simulink library "MIL_Test"  (Simulink 7.0)
values from neighbouring files (symbols this model uses):
  TID = min('TI' == AFT(1:2))    [PAS_callback.m]    (also in PSTID_callback.m = [block '/TID'])
undefined symbols (not defined in the file or in its folder): getdatatypespecs, slcm, StepSize
libraries: simulink x71, MIL_Test x6
(part 4 of 11)

== system MIL_Test/Validation Function/Feature extraction/Time @ sig = x/Relative tolerance ==
  sig : Inport  OutDataType=sfix(16)  OutScaling=2^0
  ref : Inport  Port=2  OutDataType=sfix(16)  OutScaling=2^0
  Abs : Abs
  Abs1 : Abs
  Add : Sum  Inputs=+-  OutDataType=sfix(16)  OutScaling=2^-10
  Divide1 : Product  Inputs=**/  OutDataType=sfix(16)  OutScaling=2^-10
  Max : Constant  Value=100  OutDataType=sfix(16)  OutScaling=2^0
  Relational Operator : RelationalOperator  Operator=<=  LogicOutDataTypeMode=boolean
  Relative Tolerance : Constant  Value=0.0001  OutDataType=sfix(16)  OutScaling=2^0
  sig == ref : Outport  OutDataType=sfix(16)  OutScaling=2^0
  wires:
  Abs1/1 -> Divide1/1
  Relational Operator/1 -> sig == ref/1
  Relative Tolerance/1 -> Divide1/2
  Max/1 -> Divide1/3
  Divide1/1 -> Relational Operator/2
  ref/1 -> Abs1/1, Add/2
  sig/1 -> Add/1
  Add/1 -> Abs/1
  Abs/1 -> Relational Operator/1

== system MIL_Test/Validation Function/Feature extraction/Time since signal constant/Detect constant ==
  Signal : Inport  OutDataType=sfix(16)  OutScaling=2^0
  Clock : Clock
      settings: Decimation=10
  Constant1 : Constant  Value=0  OutDataTypeMode=boolean  OutDataType=sfix(16)  OutScaling=2^0
  Memory : Memory
  Relative tolerance : Subsystem
  Switch : Switch  Criteria=u2 > Threshold
  Constant : Outport  OutDataType=sfix(16)  OutScaling=2^0
  wires:
  Switch/1 -> Constant/1
  Relative tolerance/1(sig == ref) -> Switch/1
  Clock/1 -> Switch/2
  Constant1/1 -> Switch/3
  Memory/1 -> Relative tolerance/2(ref)
  Signal/1 -> Relative tolerance/1(sig), Memory/1

== system MIL_Test/Validation Function/TODO/<system name>/<Requirement name> ==
  InOut Bus : Inport  OutDataType=sfix(16)  OutScaling=2^0
  <Assertions name> : Subsystem  Description=Assertions template. Create a new assertions block from this template.
  <Preconditions name> : Subsystem  Description=Preconditions template. Create new preconditions blocks using this template.
  Bus Creator : BusCreator  Inputs=1
  Test Info : Outport  OutDataType=sfix(16)  OutScaling=2^0
  wires:
  <Preconditions name>/1(Activate) -> <Assertions name>/1(Precond)
  Bus Creator/1 -> Test Info/1
  <Assertions name>/1(VF info) -> Bus Creator/1
  InOut Bus/1 -> <Preconditions name>/1(InOut Bus), <Assertions name>/2(InOut Bus)

== system MIL_Test/Validation Function/TODO/Assertions/Fault info ==
  Local Verdict : Inport  OutDataType=sfix(16)  OutScaling=2^0
  Expected lower limit : Inport  Port=2  OutDataType=sfix(16)  OutScaling=2^0
  Expected upper limit : Inport  Port=3  OutDataType=sfix(16)  OutScaling=2^0
  Actual Data : Inport  Port=4  OutDataType=sfix(16)  OutScaling=2^0
  Enable : EnablePort
  Assertions : Constant  Value=Ass  OutDataType=sfix(16)  OutScaling=2^0
  Bus Creator : BusCreator  Inputs=5
  Bus Creator1 : BusCreator  Inputs=3
  Data Type Conversion{,1..3} (4 alike) : DataTypeConversion  OutDataType=sfix(16)  OutScaling=2^0
  Preconditions : Constant  Value=Pre  OutDataType=sfix(16)  OutScaling=2^0
  Requirement : Constant  Value=Req  OutDataType=sfix(16)  OutScaling=2^0
  VF info : Outport  OutDataType=sfix(16)  OutScaling=2^0  OutputWhenDisabled=reset  InitialOutput=[2]
  wires:
  Requirement/1 -> Bus Creator1/3  "Requirement"
  Preconditions/1 -> Bus Creator1/2  "Preconditions"
  Assertions/1 -> Bus Creator1/1  "Assertions"
  Data Type Conversion3/1 -> Bus Creator/4  "Actual data"
  Data Type Conversion2/1 -> Bus Creator/3  "Expected upper limit"
  Data Type Conversion1/1 -> Bus Creator/2  "Expected lower limit"
  Data Type Conversion/1 -> Bus Creator/1  "Local verdict"
  Local Verdict/1 -> Data Type Conversion/1  "Local verdict"
  Expected upper limit/1 -> Data Type Conversion2/1  "Expected upper limit"
  Expected lower limit/1 -> Data Type Conversion1/1  "Expected lower limit"
  Actual Data/1 -> Data Type Conversion3/1  "Actual Data"
  Bus Creator1/1 -> Bus Creator/5  "Source"
  Bus Creator/1 -> VF info/1

== system MIL_Test/Validation Function/TODO/Assertions/Signal comparison ==
  Bound : Subsystem  mask(Bound){cm=>=, Lower=0, Upper=1}
      mask prompts: cm "Comparison method:"; Upper "Mask Parameter 3:"
      mask help:
      | Compare a signal with a reference using the specified comparison method.
      |
      | Output verdict V and lower (LL) and upper (UL) limits for reporting.
      |
      | For '==' or '~=' use "Range - Gap"
      mask init:
      | set_param([get_param(gcb,'Parent') '/' get_param(gcb,'Name') '/Relational Operator'],'Operator',get_param(gcb,'cm'));
      | set_param(gcb,'Upper',num2str(uint8(max(get_param([get_param(gcb,'Parent') '/' get_param(gcb,'Name') '/Relational Operator'],'Operator') == '>'))));
      | set_param(gcb,'Lower',num2str(uint8(max(get_param([get_param(gcb,'Parent') '/' get_param(gcb,'Name') '/Relational Operator'],'Operator') == '<'))));
      mask StyleString: popup(>|>=|<=|<),edit,edit
      mask Display:
      | port_label('output', 1, 'V');
      | port_label('output', 2, 'LL');
      | port_label('output', 3, 'UL');
      | port_label('input', 1, 'Sig');
      | port_label('input', 2, 'Ref');
      | text(0.05,0.5,get_param(get_param([get_param(gcb,'Parent') '/' get_param(gcb,'Name') '/Relational Operator'],'handle'),'Operator'));
  Range - Gap Absolute tolerance : Subsystem  mask(Range - Gap Absolute Tolerance){GorR=Range, AbsoluteTolerance=100}
      mask prompts: GorR "Use range or gap"; AbsoluteTolerance "Absolute Tolerance"
      mask help:
      | Check that a signal stays inside a range or outside a gap around a reference signal. Specify the range or the gap absolute to the reference signal.
      |
      | Output verdict V and lower (LL) and upper (UL) limits for reporting.
      mask init: same as MIL_Test/Test Data/Signal comparison/Range - Gap Relative tolerance Precond
      mask StyleString: popup(Range|Gap  ),edit
      mask Display:
      | port_label('output',1,'V');
      | port_label('output',2,'LL');
      | port_label('output',3,'UL');
      | port_label('input',1,'Sig');
      | port_label('input',2,'Ref');
      | text(0.40,0.53,'+');
      | text(0.415,0.46,'-');
      | text(0.5,0.5,num2str(AbsoluteTolerance));
      | text(0.05,0.5,helpVariable2);
  Range - Gap Relative tolerance : Subsystem  mask(Range - Gap Relative Tolerance){GorR=Range, RelativeTolerance=1}
      mask prompts: GorR "Use range or gap"; RelativeTolerance "Relative Tolerance in Percent"
      mask help:
      | Check that a signal stays inside a range or outside a gap around a reference signal. Specify the range or the gap relative to the reference signal.
      |
      | Output verdict V and lower (LL) and upper (UL) limits for reporting.
      mask init: same as MIL_Test/Test Data/Signal comparison/Range - Gap Relative tolerance Precond
      mask StyleString: popup(Range|Gap  ),edit
      mask Display:
      | port_label('output',1,'V');
      | port_label('output',2,'LL');
      | port_label('output',3,'UL');
      | port_label('input',1,'Sig');
      | port_label('input',2,'Ref');
      | text(0.425,0.5,[num2str(RelativeTolerance) ' %']);
      | text(0.05,0.5,helpVariable2);
  Range - Gap Tolerance range : Subsystem  mask(Range - Gap Tolerance range){GorR=Range}
      mask prompts: GorR "Use range or gap"
      mask help:
      | Check that a signal stays inside a dynamically specified value range.
      |
      | Output verdict V and lower (LL) and upper (UL) limits for reporting.
      mask init:
      | if max(get_param(gcb,'GorR') == ' ') % Gap
      |     helpVariable1 = '<=';
      | else % Range
      |     helpVariable1 = '>=';
      | end
      | set_param([get_param(gcb,'Parent') '/' get_param(gcb,'Name') '/Relational Operator'],'Operator',helpVariable1);
      | clear helpVariable1;
      mask StyleString: popup(Range|Gap  )
      mask Display:
      | port_label('output',1,'V');
      | port_label('output',2,'LL');
      | port_label('output',3,'UL');
      | port_label('input',1,'Sig');
      | port_label('input',2,'Lower Bound');
      | port_label('input',3,'Upper Bound');
      | patch(0.05+[0.3 0.7 0.7 0.3],-0.05+[0.8 0.8 0.9 0.9],[1 1 1]*double(not(max(get_param(gcb,'GorR') == ' '))));
      | patch(0.05+[0.3 0.7 0.7 0.3],-0.05+[0.9 0.9 0.95 0.95],[1 1 1]*double(max(get_param(gcb,'GorR') == ' ')));
      | patch(0.05+[0.3 0.7 0.7 0.3],-0.05+[0.75 0.75 0.8 0.8],[1 1 1]*double(max(get_param(gcb,'GorR') == ' ')));
      | patch(0.05+[0.25 0.25 0.8 0.8 0.26 0.26],[0.95 0.65 0.65 0.66 0.66 0.95],[0 0 0]);
      | patch(0.033+[0.27 0.22 0.23 0.27 0.31 0.32 0.27],0.02+[0.95 0.85 0.85 0.89 0.85 0.85 0.95],[0 0 0]);
      | patch(0.17+[0.7 0.6 0.6 0.65 0.6 0.6 0.7],-0.043+[0.7 0.63 0.64 0.7 0.76 0.77 0.7],[0 0 0]);

== system MIL_Test/Validation Function/TODO/Model Info/EmptySubsystem ==

== system MIL_Test/Validation Function/TODO/Preconditions/Signal comparison ==
  Bound : Subsystem  mask(Bound){cm=>=}
      mask prompts: cm "Comparison method:"
      mask help:
      | Compare a signal with a reference using the specified comparison method.
      |
      | For '==' or '~=' use "Range - Gap"
      mask init:
      | bp = get_param(gcbh,'Parent');
      | bn = get_param(gcbh,'Name');
      | set_param([bp '/' bn '/RelOp'],'Operator',get_param(gcbh,'cm'));
      mask StyleString: popup(>|>=|<=|<)
      mask Display:
      | port_label('output', 1, 'A');
      | port_label('input', 1, 'Sig');
      | port_label('input', 2, 'Ref');
      | text(0.05,0.5,get_param(get_param([get_param(gcb,'Parent') '/' get_param(gcb,'Name') '/RelOp'],'handle'),'Operator'));
  Range - Gap Absolute tolerance : Subsystem  mask(Range - Gap Absolute Tolerance){GorR=Range, AbsoluteTolerance=100}
      mask prompts: GorR "Use range or gap"; AbsoluteTolerance "Absolute Tolerance"
      mask help: Check that a signal stays inside a range or outside a gap around a reference signal. Specify the range or the gap absolute to the reference signal.
      mask init:
      | if max(get_param(gcb,'GorR') == ' ') % Gap
      |     helpVariable1 = '>=';
      |     helpVariable2 = '~=';
      | else % Range
      |     helpVariable1 = '<=';
      |     helpVariable2 = '==';
      | end
      | set_param([get_param(gcb,'Parent') '/' get_param(gcb,'Name') '/Relational Operator'],'Operator',helpVariable1);
      | set_param(gcb,'Op',helpVariable2);
      | clear helpVariable1;
      mask StyleString: popup(Range|Gap  ),edit
      mask Display:
      | port_label('output',1,'A');
      | port_label('input',1,'Sig');
      | port_label('input',2,'Ref');
      | text(0.40,0.53,'+');
      | text(0.415,0.46,'-');
      | text(0.5,0.5,num2str(AbsoluteTolerance));
      | text(0.05,0.5,helpVariable2);
  Range - Gap Relative tolerance : Subsystem  mask(Range - Gap Relative Tolerance){GorR=Range, RelativeTolerance=1}
      mask prompts: GorR "Use range or gap"; RelativeTolerance "Relative Tolerance in Percent"
      mask help: Check that a signal stays inside a range or outside a gap around a reference signal. Specify the range or the gap relative to the reference signal.
      mask init: same as MIL_Test/Test Data/Signal comparison/Range - Gap Relative tolerance Precond
      mask StyleString: popup(Range|Gap  ),edit
      mask Display:
      | port_label('output',1,'A');
      | port_label('input',1,'Sig');
      | port_label('input',2,'Ref');
      | text(0.425,0.5,[num2str(RelativeTolerance) ' %']);
      | text(0.05,0.5,helpVariable2);
  Range - Gap Tolerance range : Subsystem  mask(Range - Gap Tolerance range){GorR=Range}
      mask prompts: GorR "Use range or gap"
      mask help: Check that a signal stays inside a dynamically specified value range.
      mask init: same as MIL_Test/Validation Function/TODO/Assertions/Signal comparison/Range - Gap Tolerance range
      mask StyleString: popup(Range|Gap  )
      mask Display:
      | port_label('output',1,'A');
      | port_label('input',1,'Sig');
      | port_label('input',2,'Lower Bound');
      | port_label('input',3,'Upper Bound');
      | patch(0.05+[0.3 0.7 0.7 0.3],-0.05+[0.8 0.8 0.9 0.9],[1 1 1]*double(not(max(get_param(gcb,'GorR') == ' '))));
      | patch(0.05+[0.3 0.7 0.7 0.3],-0.05+[0.9 0.9 0.95 0.95],[1 1 1]*double(max(get_param(gcb,'GorR') == ' ')));
      | patch(0.05+[0.3 0.7 0.7 0.3],-0.05+[0.75 0.75 0.8 0.8],[1 1 1]*double(max(get_param(gcb,'GorR') == ' ')));
      | patch(0.05+[0.25 0.25 0.8 0.8 0.26 0.26],[0.95 0.65 0.65 0.66 0.66 0.95],[0 0 0]);
      | patch(0.033+[0.27 0.22 0.23 0.27 0.31 0.32 0.27],0.02+[0.95 0.85 0.85 0.89 0.85 0.85 0.95],[0 0 0]);
      | patch(0.17+[0.7 0.6 0.6 0.65 0.6 0.6 0.7],-0.043+[0.7 0.63 0.64 0.7 0.76 0.77 0.7],[0 0 0]);

== system MIL_Test/Validation Function/TODO/Validation FunctionsTemplate/Arbitration ==
  In1 : Inport  OutDataType=sfix(16)  OutScaling=2^0
  Collect Verdicts : MinMax  Inputs=3  OutDataType=sfix(16)  OutScaling=2^0
  Memory : Memory  Orientation=left  X0=2
  Out1 : Outport  OutDataType=sfix(16)  OutScaling=2^0
  wires:
  Collect Verdicts/1 -> Memory/1, Out1/1
  In1/1 -> Collect Verdicts/1
  Memory/1 -> Collect Verdicts/3

== system MIL_Test/Validation Function/TODO/Validation FunctionsTemplate/Datatype conversion ==
  InOutBus : Inport  OutDataType=sfix(16)  OutScaling=2^0
  Bus Creator{,1..5} (6 alike) : BusCreator  Inputs=2
  Bus Selector : BusSelector  OutputSignals=Inputs,Outputs
  Bus Selector1 : BusSelector  OutputSignals=v_Fzg,signal2
  Bus Selector2 : BusSelector  OutputSignals=signal1,signal2
  Bus Selector3 : BusSelector  OutputSignals=phi_Acc,phi_Brake
  Bus Selector4 : BusSelector  OutputSignals=T_des_Drive,T_des_Brake
  Bus Selector5 : BusSelector  OutputSignals=AccPedal,BrakePedal
  Data Type Conversion{,1..6} (7 alike) : DataTypeConversion  OutDataType=sfix(16)  OutScaling=2^0
  InOut Bus : Outport  OutDataType=sfix(16)  OutScaling=2^0
  wires:
  Bus Creator5/1 -> InOut Bus/1  "InOutBus"
  Bus Creator4/1 -> Bus Creator5/2  "Outputs"
  Bus Creator3/1 -> Bus Creator5/1  "Inputs"
  Bus Creator1/1 -> Bus Creator4/2
  Bus Creator/1 -> Bus Creator4/1
  Data Type Conversion/1 -> Bus Creator3/1  "v_Fzg"
  Bus Creator2/1 -> Bus Creator3/2  "signal2"
  Data Type Conversion2/1 -> Bus Creator2/2  "phi_Brake"
  Data Type Conversion1/1 -> Bus Creator2/1  "phi_Acc"
  Data Type Conversion6/1 -> Bus Creator1/2  "BrakePedal"
  Data Type Conversion5/1 -> Bus Creator1/1  "AccPedal"
  Data Type Conversion4/1 -> Bus Creator/2  "T_des_Brake"
  Data Type Conversion3/1 -> Bus Creator/1  "T_des_Drive"
  Bus Selector5/2 -> Data Type Conversion6/1  "<BrakePedal>"
  Bus Selector5/1 -> Data Type Conversion5/1  "<AccPedal>"
  Bus Selector4/2 -> Data Type Conversion4/1  "<T_des_Brake>"
  Bus Selector4/1 -> Data Type Conversion3/1  "<T_des_Drive>"
  Bus Selector3/2 -> Data Type Conversion2/1  "<phi_Brake>"
  Bus Selector3/1 -> Data Type Conversion1/1  "<phi_Acc>"
  Bus Selector1/1 -> Data Type Conversion/1  "<v_Fzg>"
  Bus Selector2/2 -> Bus Selector5/1  "<signal2>"
  Bus Selector2/1 -> Bus Selector4/1  "<signal1>"
  Bus Selector1/2 -> Bus Selector3/1  "<signal2>"
  Bus Selector/2 -> Bus Selector2/1  "<Outputs>"
  Bus Selector/1 -> Bus Selector1/1  "<Inputs>"
  InOutBus/1 -> Bus Selector/1

== system MIL_Test/Validation Function/TODO/Validation FunctionsTemplate/Requirement ==
  InOut Bus : Inport  OutDataType=sfix(16)  OutScaling=2^0
  Assertions : Subsystem  TreatAsAtomicUnit=on
  Bus Creator : BusCreator  Inputs=1
  Preconditions : Subsystem
  Validation Information : Outport  OutDataType=sfix(16)  OutScaling=2^0
  wires:
  Assertions/1(VF info) -> Bus Creator/1
  Bus Creator/1 -> Validation Information/1
  InOut Bus/1 -> Preconditions/1(InOut Bus), Assertions/2(InOut Bus)
  Preconditions/1(Activate) -> Assertions/1(Activate)

== system MIL_Test/Validation Function/TODO/Validation FunctionsTemplate/Requirement2 ==
  InOut Bus : Inport  OutDataType=sfix(16)  OutScaling=2^0
  Assertions : Subsystem  TreatAsAtomicUnit=on
  Bus Creator : BusCreator  Inputs=1
  Preconditions : Subsystem
  Validation Information : Outport  OutDataType=sfix(16)  OutScaling=2^0
  wires:
  Preconditions/1(Activate) -> Assertions/1(Activate)
  InOut Bus/1 -> Assertions/2(InOut Bus), Preconditions/1(InOut Bus)
  Bus Creator/1 -> Validation Information/1
  Assertions/1(VF info) -> Bus Creator/1

== system MIL_Test/Validation Function/Test Evaluation Architecture/<system name>/<Requirement name> ==
  InOut Bus : Inport  OutDataType=sfix(16)  OutScaling=2^0
  <Assertions name> : Subsystem  Description=Assertions template. Create a new assertions block from this template.
  <Preconditions name> : Subsystem  Description=Preconditions template. Create new preconditions blocks using this template.
  Bus Creator : BusCreator  Inputs=1
  Test Info : Outport  OutDataType=sfix(16)  OutScaling=2^0
  wires:
  InOut Bus/1 -> <Assertions name>/2(InOut Bus), <Preconditions name>/1(InOut Bus)
  <Assertions name>/1(VF info) -> Bus Creator/1
  Bus Creator/1 -> Test Info/1
  <Preconditions name>/1(Activate) -> <Assertions name>/1(Precond)

== system MIL_Test/Validation Function/Test Evaluation Architecture/<system name>/Arbitration ==
  In1 : Inport  OutDataType=sfix(16)  OutScaling=2^0
  Collect Verdicts : MinMax  Inputs=2  OutDataType=sfix(16)  OutScaling=2^0
  Memory : Memory  Orientation=left  X0=2
  Out1 : Outport  OutDataType=sfix(16)  OutScaling=2^0
  wires:
  Memory/1 -> Collect Verdicts/2
  Collect Verdicts/1 -> Memory/1, Out1/1
  In1/1 -> Collect Verdicts/1

== system MIL_Test/Test Control/Test Control Architecture/Connection Helpers/TestControl for  TestCases Sequencing NoMask/IF Signal@SimStopTime for TC = value1 ==
  Signal : Inport  OutDataType=sfix(16)  OutScaling=2^0
  Current Sim StopTime : Constant  Value=currentStopTime  OutDataType=sfix(16)  OutScaling=2^0
  If : If  IfExpression=u1 ~= 1
  Model Info : simulink/Model-Wide Utilities/Model Info  SystemSampleTime=-1  InitialBlockCM=None  BlockCM=None  Frame=on  DisplayStringWithTags=|  HorizontalTextAlignment=Center  LeftAlignmentValue=0.5  SourceBlockDiagram=MIL_Test  TagMaxNumber=20
      | Flag Fullfillment = 1, then condition is true 
      | Flag Fullfillment = 0, then condition is false
  if Signal@t for TC = pass : Subsystem
  "if false, then  TC4 for 200" : Subsystem
  "if true, then  TC2 for 400" : Subsystem
  Fulfillment : Outport  OutDataType=sfix(16)  OutScaling=2^0
  wires:
  Current Sim StopTime/1 -> if Signal@t for TC = pass/1(@time)
  Signal/1 -> if Signal@t for TC = pass/2(Signal1)
  If/1 -> "if false, then  TC4 for 200"/Action
  If/2 -> "if true, then  TC2 for 400"/Action
  if Signal@t for TC = pass/1(Control Seq1) -> Fulfillment/1

== system MIL_Test/Test Control/Test Control Architecture/Connection Helpers/TestControl for  TestCases Sequencing NoMask/IF signal @[timeUp, timeDown] for TC = value1 ==
  Signal : Inport  OutDataType=sfix(16)  OutScaling=2^0
  TimeDown : Constant  Value=timeDown  OutDataType=sfix(16)  OutScaling=2^0
  TimeUp : Constant  Value=timeUp  OutDataType=sfix(16)  OutScaling=2^0
  if Signal@ [TDown,TUp]  for TC = Value : Subsystem
  Fulfillment : Outport  OutDataType=sfix(16)  OutScaling=2^0
  wires:
  TimeDown/1 -> if Signal@ [TDown,TUp]  for TC = Value/1(@timeDown)
  TimeUp/1 -> if Signal@ [TDown,TUp]  for TC = Value/2(@timeUp)
  Signal/1 -> if Signal@ [TDown,TUp]  for TC = Value/3(Signal)
  if Signal@ [TDown,TUp]  for TC = Value/1(Control Seq) -> Fulfillment/1

== system MIL_Test/Test Control/Test Control Architecture/Connection Helpers/TestControl for  TestCases Sequencing NoMask/IF signal@time for TC = value1 ==
  Signal : Inport  OutDataType=sfix(16)  OutScaling=2^0
  given Time : Constant  Value=time  OutDataType=sfix(16)  OutScaling=2^0
  if Signal@t for TC = pass : Subsystem
  Fulfillment : Outport  OutDataType=sfix(16)  OutScaling=2^0
  wires:
  given Time/1 -> if Signal@t for TC = pass/1(@time)
  Signal/1 -> if Signal@t for TC = pass/2(Signal1)
  if Signal@t for TC = pass/1(Control Seq) -> Fulfillment/1

== system MIL_Test/Test Control/Test Control Architecture/Test Control Conditions/IF Signal@SimStopTime for TC = value1/if Signal@t for TC = pass ==
  @time : Inport  OutDataType=sfix(16)  OutScaling=2^0
  Signal1 : Inport  Port=2  OutDataType=sfix(16)  OutScaling=2^0
  ClockAtEnd : Clock
      settings: Decimation=10
  Relational Operator1 : RelationalOperator  LogicOutDataTypeMode=boolean
  check in range : Subsystem  TreatAsAtomicUnit=on
  Control Seq1 : Outport  OutDataType=sfix(16)  OutScaling=2^0
  wires:
  Relational Operator1/1 -> check in range/Enable, check in range/1(@[time])
  check in range/1(Control Seq) -> Control Seq1/1
  Signal1/1 -> check in range/2(Signal)
  @time/1 -> Relational Operator1/2
  ClockAtEnd/1 -> Relational Operator1/1

== system MIL_Test/Test Control/Test Control Architecture/Test Control Conditions/IF Signal@SimStopTime for TC = value1/if false, then  TC4 for 200 ==
  Action Port : ActionPort
  Embedded MATLAB Function : Stateflow chart

== system MIL_Test/Test Control/Test Control Architecture/Test Control Conditions/IF Signal@SimStopTime for TC = value1/if true, then  TC2 for 400 ==
  Action Port : ActionPort
  Embedded MATLAB Function : Stateflow chart

== system MIL_Test/Test Control/Test Control Architecture/Test Control Conditions/IF signal @[timeUp, timeDown] for TC = value1/if Signal@ [TDown,TUp]  for TC = Value ==
  @timeDown : Inport  OutDataType=sfix(16)  OutScaling=2^0
  @timeUp : Inport  Port=2  OutDataType=sfix(16)  OutScaling=2^0
  Signal : Inport  Port=3  OutDataType=sfix(16)  OutScaling=2^0
  ClockDuring : Clock
      settings: Decimation=10
  Logical Operator1 : Logic  AllPortsSameDT=off  OutDataTypeMode=boolean
  Relational Operator1 : RelationalOperator  LogicOutDataTypeMode=boolean
  Relational Operator2 : RelationalOperator  Operator=<=  LogicOutDataTypeMode=boolean
  check in range : Subsystem  TreatAsAtomicUnit=on
  Control Seq : Outport  OutDataType=sfix(16)  OutScaling=2^0
  wires:
  check in range/1(Control Seq) -> Control Seq/1
  Signal/1 -> check in range/2(Signal)
  Logical Operator1/1 -> check in range/Enable, check in range/1(@[time])
  Relational Operator2/1 -> Logical Operator1/2
  Relational Operator1/1 -> Logical Operator1/1
  @timeUp/1 -> Relational Operator2/2
  @timeDown/1 -> Relational Operator1/2
  ClockDuring/1 -> Relational Operator2/1, Relational Operator1/1

== system MIL_Test/Test Control/Test Control Architecture/Test Control Conditions/IF signal@time for TC = value1/if Signal@t for TC = pass ==
  @time : Inport  OutDataType=sfix(16)  OutScaling=2^0
  Signal1 : Inport  Port=2  OutDataType=sfix(16)  OutScaling=2^0
  ClockAtTime : Clock
      settings: Decimation=10
  Relational Operator1 : RelationalOperator  LogicOutDataTypeMode=boolean
  check in range : Subsystem  TreatAsAtomicUnit=on
  Control Seq : Outport  OutDataType=sfix(16)  OutScaling=2^0
  wires:
  check in range/1(Control Seq) -> Control Seq/1
  Signal1/1 -> check in range/2(Signal)
  Relational Operator1/1 -> check in range/Enable, check in range/1(@[time])
  @time/1 -> Relational Operator1/2
  ClockAtTime/1 -> Relational Operator1/1

== system MIL_Test/Test Control/Test Control Architecture/Test Control Conditions/IF signal@time1/if Signal@t for TC = pass ==
  @time : Inport  OutDataType=sfix(16)  OutScaling=2^0
  Signal1 : Inport  Port=2  OutDataType=sfix(16)  OutScaling=2^0
  Clock : Clock
      settings: Decimation=10
  Relational Operator1 : RelationalOperator  LogicOutDataTypeMode=boolean
  check in range : Subsystem  TreatAsAtomicUnit=on
  Control Seq : Outport  OutDataType=sfix(16)  OutScaling=2^0
  wires:
  Relational Operator1/1 -> check in range/Enable, check in range/1(@[time])
  check in range/1(Control Seq) -> Control Seq/1
  Signal1/1 -> check in range/2(Signal)
  @time/1 -> Relational Operator1/2
  Clock/1 -> Relational Operator1/1

== system MIL_Test/Test Control/Test Control Architecture/Test Control Conditions/IF signal@time1/if false, then  TC4 for 200 ==
  Action Port : ActionPort
  Embedded MATLAB Function : Stateflow chart

== system MIL_Test/Test Control/Test Control Architecture/Test Control Conditions/IF signal@time1/if true, then  TC2 for 400 ==
  Action Port : ActionPort
  Embedded MATLAB Function : Stateflow chart

== system MIL_Test/Test Data/Feature generation/Generate  local maximum  with given slope/Limited Ramp Increasing/Enabled Subsystem1 ==
  In2 : Inport  OutDataType=sfix(16)  OutScaling=2^0
  Enable : EnablePort  StatesWhenEnabling=reset
  MaxValue1 : Outport  OutDataType=sfix(16)  OutScaling=2^0  InitialOutput=[0]
  wires:
  In2/1 -> MaxValue1/1

== system MIL_Test/Test Data/Feature generation/Generate timed limited decrease/Subsystem/Subsystem1 ==
  In1 : Inport  OutDataType=sfix(16)  OutScaling=2^0
  In2 : Inport  Port=2  OutDataType=sfix(16)  OutScaling=2^0
  In3 : Inport  Port=3  OutDataType=sfix(16)  OutScaling=2^0
  Output1 : Sum  Inputs=|+-+  OutDataType=sfix(16)  OutScaling=2^0  SaturateOnIntegerOverflow=on  InputSameDT=on
  RO : RelationalOperator  Operator=<  LogicOutDataTypeMode=boolean
  Switch : Switch  Criteria=u2 > Threshold
  Out1 : Outport  OutDataType=sfix(16)  OutScaling=2^0
  wires:
  In3/1 -> Output1/3
  Output1/1 -> Switch/1
  RO/1 -> Switch/2
  Switch/1 -> Out1/1
  In2/1 -> RO/1, Output1/1, Switch/3  "U(k)"
  In1/1 -> RO/2, Output1/2

== system MIL_Test/Test Data/Feature generation/Generate timed limited decrease/Subsystem/Subsystem10 ==
  In1 : Inport  OutDataType=sfix(16)  OutScaling=2^0
  In2 : Inport  Port=2  OutDataType=sfix(16)  OutScaling=2^0
  In3 : Inport  Port=3  OutDataType=sfix(16)  OutScaling=2^0
  Output1 : Sum  Inputs=|+-+  OutDataType=sfix(16)  OutScaling=2^0  SaturateOnIntegerOverflow=on  InputSameDT=on
  RO : RelationalOperator  Operator=<  LogicOutDataTypeMode=boolean
  Switch : Switch  Criteria=u2 > Threshold
  Out1 : Outport  OutDataType=sfix(16)  OutScaling=2^0
  wires:
  In3/1 -> Output1/3
  Output1/1 -> Switch/1
  RO/1 -> Switch/2
  Switch/1 -> Out1/1
  In2/1 -> RO/1, Output1/1, Switch/3  "U(k)"
  In1/1 -> RO/2, Output1/2

== system MIL_Test/Test Data/Feature generation/Generate timed limited decrease/Subsystem/Subsystem11 ==
  In1 : Inport  OutDataType=sfix(16)  OutScaling=2^0
  In2 : Inport  Port=2  OutDataType=sfix(16)  OutScaling=2^0
  In3 : Inport  Port=3  OutDataType=sfix(16)  OutScaling=2^0
  Output1 : Sum  Inputs=|+-+  OutDataType=sfix(16)  OutScaling=2^0  SaturateOnIntegerOverflow=on  InputSameDT=on
  RO : RelationalOperator  Operator=<  LogicOutDataTypeMode=boolean
  Switch : Switch  Criteria=u2 > Threshold
  Out1 : Outport  OutDataType=sfix(16)  OutScaling=2^0
  wires:
  In3/1 -> Output1/3
  Output1/1 -> Switch/1
  RO/1 -> Switch/2
  Switch/1 -> Out1/1
  In2/1 -> RO/1, Output1/1, Switch/3  "U(k)"
  In1/1 -> RO/2, Output1/2

== system MIL_Test/Test Data/Feature generation/Generate timed limited decrease/Subsystem/Subsystem12 ==
  In1 : Inport  OutDataType=sfix(16)  OutScaling=2^0
  In2 : Inport  Port=2  OutDataType=sfix(16)  OutScaling=2^0
  In3 : Inport  Port=3  OutDataType=sfix(16)  OutScaling=2^0
  Output1 : Sum  Inputs=|+-+  OutDataType=sfix(16)  OutScaling=2^0  SaturateOnIntegerOverflow=on  InputSameDT=on
  RO : RelationalOperator  Operator=<  LogicOutDataTypeMode=boolean
  Switch : Switch  Criteria=u2 > Threshold
  Out1 : Outport  OutDataType=sfix(16)  OutScaling=2^0
  wires:
  In3/1 -> Output1/3
  Output1/1 -> Switch/1
  RO/1 -> Switch/2
  Switch/1 -> Out1/1
  In2/1 -> RO/1, Output1/1, Switch/3  "U(k)"
  In1/1 -> RO/2, Output1/2

== system MIL_Test/Test Data/Feature generation/Generate timed limited decrease/Subsystem/Subsystem13 ==
  In1 : Inport  OutDataType=sfix(16)  OutScaling=2^0
  In2 : Inport  Port=2  OutDataType=sfix(16)  OutScaling=2^0
  In3 : Inport  Port=3  OutDataType=sfix(16)  OutScaling=2^0
  Output1 : Sum  Inputs=|+-+  OutDataType=sfix(16)  OutScaling=2^0  SaturateOnIntegerOverflow=on  InputSameDT=on
  RO : RelationalOperator  Operator=<  LogicOutDataTypeMode=boolean
  Switch : Switch  Criteria=u2 > Threshold
  Out1 : Outport  OutDataType=sfix(16)  OutScaling=2^0
  wires:
  In3/1 -> Output1/3
  Output1/1 -> Switch/1
  RO/1 -> Switch/2
  Switch/1 -> Out1/1
  In2/1 -> RO/1, Output1/1, Switch/3  "U(k)"
  In1/1 -> RO/2, Output1/2

== system MIL_Test/Test Data/Feature generation/Generate timed limited decrease/Subsystem/Subsystem14 ==
  In1 : Inport  OutDataType=sfix(16)  OutScaling=2^0
  In2 : Inport  Port=2  OutDataType=sfix(16)  OutScaling=2^0
  In3 : Inport  Port=3  OutDataType=sfix(16)  OutScaling=2^0
  Output1 : Sum  Inputs=|+-+  OutDataType=sfix(16)  OutScaling=2^0  SaturateOnIntegerOverflow=on  InputSameDT=on
  RO : RelationalOperator  Operator=<  LogicOutDataTypeMode=boolean
  Switch : Switch  Criteria=u2 > Threshold
  Out1 : Outport  OutDataType=sfix(16)  OutScaling=2^0
  wires:
  In3/1 -> Output1/3
  Output1/1 -> Switch/1
  RO/1 -> Switch/2
  Switch/1 -> Out1/1
  In2/1 -> RO/1, Output1/1, Switch/3  "U(k)"
  In1/1 -> RO/2, Output1/2

== system MIL_Test/Test Data/Feature generation/Generate timed limited decrease/Subsystem/Subsystem15 ==
  In1 : Inport  OutDataType=sfix(16)  OutScaling=2^0
  In2 : Inport  Port=2  OutDataType=sfix(16)  OutScaling=2^0
  In3 : Inport  Port=3  OutDataType=sfix(16)  OutScaling=2^0
  Output1 : Sum  Inputs=|+-+  OutDataType=sfix(16)  OutScaling=2^0  SaturateOnIntegerOverflow=on  InputSameDT=on
  RO : RelationalOperator  Operator=<  LogicOutDataTypeMode=boolean
  Switch : Switch  Criteria=u2 > Threshold
  Out1 : Outport  OutDataType=sfix(16)  OutScaling=2^0
  wires:
  In3/1 -> Output1/3
  Output1/1 -> Switch/1
  RO/1 -> Switch/2
  Switch/1 -> Out1/1
  In2/1 -> RO/1, Output1/1, Switch/3  "U(k)"
  In1/1 -> RO/2, Output1/2

== system MIL_Test/Test Data/Feature generation/Generate timed limited decrease/Subsystem/Subsystem16 ==
  In1 : Inport  OutDataType=sfix(16)  OutScaling=2^0
  In2 : Inport  Port=2  OutDataType=sfix(16)  OutScaling=2^0
  In3 : Inport  Port=3  OutDataType=sfix(16)  OutScaling=2^0
  Output1 : Sum  Inputs=|+-+  OutDataType=sfix(16)  OutScaling=2^0  SaturateOnIntegerOverflow=on  InputSameDT=on
  RO : RelationalOperator  Operator=<  LogicOutDataTypeMode=boolean
  Switch : Switch  Criteria=u2 > Threshold
  Out1 : Outport  OutDataType=sfix(16)  OutScaling=2^0
  wires:
  In3/1 -> Output1/3
  Output1/1 -> Switch/1
  RO/1 -> Switch/2
  Switch/1 -> Out1/1
  In2/1 -> RO/1, Output1/1, Switch/3  "U(k)"
  In1/1 -> RO/2, Output1/2

== system MIL_Test/Test Data/Feature generation/Generate timed limited decrease/Subsystem/Subsystem17 ==
  In1 : Inport  OutDataType=sfix(16)  OutScaling=2^0
  In2 : Inport  Port=2  OutDataType=sfix(16)  OutScaling=2^0
  In3 : Inport  Port=3  OutDataType=sfix(16)  OutScaling=2^0
  Output1 : Sum  Inputs=|+-+  OutDataType=sfix(16)  OutScaling=2^0  SaturateOnIntegerOverflow=on  InputSameDT=on
  RO : RelationalOperator  Operator=<  LogicOutDataTypeMode=boolean
  Switch : Switch  Criteria=u2 > Threshold
  Out1 : Outport  OutDataType=sfix(16)  OutScaling=2^0
  wires:
  In3/1 -> Output1/3
  Output1/1 -> Switch/1
  RO/1 -> Switch/2
  Switch/1 -> Out1/1
  In2/1 -> RO/1, Output1/1, Switch/3  "U(k)"
  In1/1 -> RO/2, Output1/2

== system MIL_Test/Test Data/Feature generation/Generate timed limited decrease/Subsystem/Subsystem18 ==
  In1 : Inport  OutDataType=sfix(16)  OutScaling=2^0
  In2 : Inport  Port=2  OutDataType=sfix(16)  OutScaling=2^0
  In3 : Inport  Port=3  OutDataType=sfix(16)  OutScaling=2^0
  Output1 : Sum  Inputs=|+-+  OutDataType=sfix(16)  OutScaling=2^0  SaturateOnIntegerOverflow=on  InputSameDT=on
  RO : RelationalOperator  Operator=<  LogicOutDataTypeMode=boolean
  Switch : Switch  Criteria=u2 > Threshold
  Out1 : Outport  OutDataType=sfix(16)  OutScaling=2^0
  wires:
  In3/1 -> Output1/3
  Output1/1 -> Switch/1
  RO/1 -> Switch/2
  Switch/1 -> Out1/1
  In2/1 -> RO/1, Output1/1, Switch/3  "U(k)"
  In1/1 -> RO/2, Output1/2

== system MIL_Test/Test Data/Feature generation/Generate timed limited decrease/Subsystem/Subsystem19 ==
  In1 : Inport  OutDataType=sfix(16)  OutScaling=2^0
  In2 : Inport  Port=2  OutDataType=sfix(16)  OutScaling=2^0
  In3 : Inport  Port=3  OutDataType=sfix(16)  OutScaling=2^0
  Output1 : Sum  Inputs=|+-+  OutDataType=sfix(16)  OutScaling=2^0  SaturateOnIntegerOverflow=on  InputSameDT=on
  RO : RelationalOperator  Operator=<  LogicOutDataTypeMode=boolean
  Switch : Switch  Criteria=u2 > Threshold
  Out1 : Outport  OutDataType=sfix(16)  OutScaling=2^0
  wires:
  In3/1 -> Output1/3
  Output1/1 -> Switch/1
  RO/1 -> Switch/2
  Switch/1 -> Out1/1
  In2/1 -> RO/1, Output1/1, Switch/3  "U(k)"
  In1/1 -> RO/2, Output1/2

== system MIL_Test/Test Data/Feature generation/Generate timed limited decrease/Subsystem/Subsystem2 ==
  In1 : Inport  OutDataType=sfix(16)  OutScaling=2^0
  In2 : Inport  Port=2  OutDataType=sfix(16)  OutScaling=2^0
  In3 : Inport  Port=3  OutDataType=sfix(16)  OutScaling=2^0
  Output1 : Sum  Inputs=|+-+  OutDataType=sfix(16)  OutScaling=2^0  SaturateOnIntegerOverflow=on  InputSameDT=on
  RO : RelationalOperator  Operator=<  LogicOutDataTypeMode=boolean
  Switch : Switch  Criteria=u2 > Threshold
  Out1 : Outport  OutDataType=sfix(16)  OutScaling=2^0
  wires:
  In3/1 -> Output1/3
  Output1/1 -> Switch/1
  RO/1 -> Switch/2
  Switch/1 -> Out1/1
  In2/1 -> RO/1, Output1/1, Switch/3  "U(k)"
  In1/1 -> RO/2, Output1/2

== system MIL_Test/Test Data/Feature generation/Generate timed limited decrease/Subsystem/Subsystem20 ==
  In1 : Inport  OutDataType=sfix(16)  OutScaling=2^0
  In2 : Inport  Port=2  OutDataType=sfix(16)  OutScaling=2^0
  In3 : Inport  Port=3  OutDataType=sfix(16)  OutScaling=2^0
  Output1 : Sum  Inputs=|+-+  OutDataType=sfix(16)  OutScaling=2^0  SaturateOnIntegerOverflow=on  InputSameDT=on
  RO : RelationalOperator  Operator=<  LogicOutDataTypeMode=boolean
  Switch : Switch  Criteria=u2 > Threshold
  Out1 : Outport  OutDataType=sfix(16)  OutScaling=2^0
  wires:
  In3/1 -> Output1/3
  Output1/1 -> Switch/1
  RO/1 -> Switch/2
  Switch/1 -> Out1/1
  In2/1 -> RO/1, Output1/1, Switch/3  "U(k)"
  In1/1 -> RO/2, Output1/2

== system MIL_Test/Test Data/Feature generation/Generate timed limited decrease/Subsystem/Subsystem21 ==
  In1 : Inport  OutDataType=sfix(16)  OutScaling=2^0
  In2 : Inport  Port=2  OutDataType=sfix(16)  OutScaling=2^0
  In3 : Inport  Port=3  OutDataType=sfix(16)  OutScaling=2^0
  Output1 : Sum  Inputs=|+-+  OutDataType=sfix(16)  OutScaling=2^0  SaturateOnIntegerOverflow=on  InputSameDT=on
  RO : RelationalOperator  Operator=<  LogicOutDataTypeMode=boolean
  Switch : Switch  Criteria=u2 > Threshold
  Out1 : Outport  OutDataType=sfix(16)  OutScaling=2^0
  wires:
  In3/1 -> Output1/3
  Output1/1 -> Switch/1
  RO/1 -> Switch/2
  Switch/1 -> Out1/1
  In2/1 -> RO/1, Output1/1, Switch/3  "U(k)"
  In1/1 -> RO/2, Output1/2

== system MIL_Test/Test Data/Feature generation/Generate timed limited decrease/Subsystem/Subsystem22 ==
  In1 : Inport  OutDataType=sfix(16)  OutScaling=2^0
  In2 : Inport  Port=2  OutDataType=sfix(16)  OutScaling=2^0
  In3 : Inport  Port=3  OutDataType=sfix(16)  OutScaling=2^0
  Output1 : Sum  Inputs=|+-+  OutDataType=sfix(16)  OutScaling=2^0  SaturateOnIntegerOverflow=on  InputSameDT=on
  RO : RelationalOperator  Operator=<  LogicOutDataTypeMode=boolean
  Switch : Switch  Criteria=u2 > Threshold
  Out1 : Outport  OutDataType=sfix(16)  OutScaling=2^0
  wires:
  In3/1 -> Output1/3
  Output1/1 -> Switch/1
  RO/1 -> Switch/2
  Switch/1 -> Out1/1
  In2/1 -> RO/1, Output1/1, Switch/3  "U(k)"
  In1/1 -> RO/2, Output1/2

== system MIL_Test/Test Data/Feature generation/Generate timed limited decrease/Subsystem/Subsystem23 ==
  In1 : Inport  OutDataType=sfix(16)  OutScaling=2^0
  In2 : Inport  Port=2  OutDataType=sfix(16)  OutScaling=2^0
  In3 : Inport  Port=3  OutDataType=sfix(16)  OutScaling=2^0
  Output1 : Sum  Inputs=|+-+  OutDataType=sfix(16)  OutScaling=2^0  SaturateOnIntegerOverflow=on  InputSameDT=on
  RO : RelationalOperator  Operator=<  LogicOutDataTypeMode=boolean
  Switch : Switch  Criteria=u2 > Threshold
  Out1 : Outport  OutDataType=sfix(16)  OutScaling=2^0
  wires:
  In3/1 -> Output1/3
  Output1/1 -> Switch/1
  RO/1 -> Switch/2
  Switch/1 -> Out1/1
  In2/1 -> RO/1, Output1/1, Switch/3  "U(k)"
  In1/1 -> RO/2, Output1/2

== system MIL_Test/Test Data/Feature generation/Generate timed limited decrease/Subsystem/Subsystem24 ==
  In1 : Inport  OutDataType=sfix(16)  OutScaling=2^0
  In2 : Inport  Port=2  OutDataType=sfix(16)  OutScaling=2^0
  In3 : Inport  Port=3  OutDataType=sfix(16)  OutScaling=2^0
  Output1 : Sum  Inputs=|+-+  OutDataType=sfix(16)  OutScaling=2^0  SaturateOnIntegerOverflow=on  InputSameDT=on
  RO : RelationalOperator  Operator=<  LogicOutDataTypeMode=boolean
  Switch : Switch  Criteria=u2 > Threshold
  Out1 : Outport  OutDataType=sfix(16)  OutScaling=2^0
  wires:
  In3/1 -> Output1/3
  Output1/1 -> Switch/1
  RO/1 -> Switch/2
  Switch/1 -> Out1/1
  In2/1 -> RO/1, Output1/1, Switch/3  "U(k)"
  In1/1 -> RO/2, Output1/2

== system MIL_Test/Test Data/Feature generation/Generate timed limited decrease/Subsystem/Subsystem25 ==
  In1 : Inport  OutDataType=sfix(16)  OutScaling=2^0
  In2 : Inport  Port=2  OutDataType=sfix(16)  OutScaling=2^0
  In3 : Inport  Port=3  OutDataType=sfix(16)  OutScaling=2^0
  Output1 : Sum  Inputs=|+-+  OutDataType=sfix(16)  OutScaling=2^0  SaturateOnIntegerOverflow=on  InputSameDT=on
  RO : RelationalOperator  Operator=<  LogicOutDataTypeMode=boolean
  Switch : Switch  Criteria=u2 > Threshold
  Out1 : Outport  OutDataType=sfix(16)  OutScaling=2^0
  wires:
  In3/1 -> Output1/3
  Output1/1 -> Switch/1
  RO/1 -> Switch/2
  Switch/1 -> Out1/1
  In2/1 -> RO/1, Output1/1, Switch/3  "U(k)"
  In1/1 -> RO/2, Output1/2

== system MIL_Test/Test Data/Feature generation/Generate timed limited decrease/Subsystem/Subsystem26 ==
  In1 : Inport  OutDataType=sfix(16)  OutScaling=2^0
  In2 : Inport  Port=2  OutDataType=sfix(16)  OutScaling=2^0
  In3 : Inport  Port=3  OutDataType=sfix(16)  OutScaling=2^0
  Output1 : Sum  Inputs=|+-+  OutDataType=sfix(16)  OutScaling=2^0  SaturateOnIntegerOverflow=on  InputSameDT=on
  RO : RelationalOperator  Operator=<  LogicOutDataTypeMode=boolean
  Switch : Switch  Criteria=u2 > Threshold
  Out1 : Outport  OutDataType=sfix(16)  OutScaling=2^0
  wires:
  In3/1 -> Output1/3
  Output1/1 -> Switch/1
  RO/1 -> Switch/2
  Switch/1 -> Out1/1
  In2/1 -> RO/1, Output1/1, Switch/3  "U(k)"
  In1/1 -> RO/2, Output1/2

== system MIL_Test/Test Data/Feature generation/Generate timed limited decrease/Subsystem/Subsystem27 ==
  In1 : Inport  OutDataType=sfix(16)  OutScaling=2^0
  In2 : Inport  Port=2  OutDataType=sfix(16)  OutScaling=2^0
  In3 : Inport  Port=3  OutDataType=sfix(16)  OutScaling=2^0
  Output1 : Sum  Inputs=|+-+  OutDataType=sfix(16)  OutScaling=2^0  SaturateOnIntegerOverflow=on  InputSameDT=on
  RO : RelationalOperator  Operator=<  LogicOutDataTypeMode=boolean
  Switch : Switch  Criteria=u2 > Threshold
  Out1 : Outport  OutDataType=sfix(16)  OutScaling=2^0
  wires:
  In3/1 -> Output1/3
  Output1/1 -> Switch/1
  RO/1 -> Switch/2
  Switch/1 -> Out1/1
  In2/1 -> RO/1, Output1/1, Switch/3  "U(k)"
  In1/1 -> RO/2, Output1/2

== system MIL_Test/Test Data/Feature generation/Generate timed limited decrease/Subsystem/Subsystem28 ==
  In1 : Inport  OutDataType=sfix(16)  OutScaling=2^0
  In2 : Inport  Port=2  OutDataType=sfix(16)  OutScaling=2^0
  In3 : Inport  Port=3  OutDataType=sfix(16)  OutScaling=2^0
  Output1 : Sum  Inputs=|+-+  OutDataType=sfix(16)  OutScaling=2^0  SaturateOnIntegerOverflow=on  InputSameDT=on
  RO : RelationalOperator  Operator=<  LogicOutDataTypeMode=boolean
  Switch : Switch  Criteria=u2 > Threshold
  Out1 : Outport  OutDataType=sfix(16)  OutScaling=2^0
  wires:
  In3/1 -> Output1/3
  Output1/1 -> Switch/1
  RO/1 -> Switch/2
  Switch/1 -> Out1/1
  In2/1 -> RO/1, Output1/1, Switch/3  "U(k)"
  In1/1 -> RO/2, Output1/2

== system MIL_Test/Test Data/Feature generation/Generate timed limited decrease/Subsystem/Subsystem29 ==
  In1 : Inport  OutDataType=sfix(16)  OutScaling=2^0
  In2 : Inport  Port=2  OutDataType=sfix(16)  OutScaling=2^0
  In3 : Inport  Port=3  OutDataType=sfix(16)  OutScaling=2^0
  Output1 : Sum  Inputs=|+-+  OutDataType=sfix(16)  OutScaling=2^0  SaturateOnIntegerOverflow=on  InputSameDT=on
  RO : RelationalOperator  Operator=<  LogicOutDataTypeMode=boolean
  Switch : Switch  Criteria=u2 > Threshold
  Out1 : Outport  OutDataType=sfix(16)  OutScaling=2^0
  wires:
  In3/1 -> Output1/3
  Output1/1 -> Switch/1
  RO/1 -> Switch/2
  Switch/1 -> Out1/1
  In2/1 -> RO/1, Output1/1, Switch/3  "U(k)"
  In1/1 -> RO/2, Output1/2

== system MIL_Test/Test Data/Feature generation/Generate timed limited decrease/Subsystem/Subsystem3 ==
  In1 : Inport  OutDataType=sfix(16)  OutScaling=2^0
  In2 : Inport  Port=2  OutDataType=sfix(16)  OutScaling=2^0
  In3 : Inport  Port=3  OutDataType=sfix(16)  OutScaling=2^0
  Output1 : Sum  Inputs=|+-+  OutDataType=sfix(16)  OutScaling=2^0  SaturateOnIntegerOverflow=on  InputSameDT=on
  RO : RelationalOperator  Operator=<  LogicOutDataTypeMode=boolean
  Switch : Switch  Criteria=u2 > Threshold
  Out1 : Outport  OutDataType=sfix(16)  OutScaling=2^0
  wires:
  In3/1 -> Output1/3
  Output1/1 -> Switch/1
  RO/1 -> Switch/2
  Switch/1 -> Out1/1
  In2/1 -> RO/1, Output1/1, Switch/3  "U(k)"
  In1/1 -> RO/2, Output1/2

== system MIL_Test/Test Data/Feature generation/Generate timed limited decrease/Subsystem/Subsystem30 ==
  In1 : Inport  OutDataType=sfix(16)  OutScaling=2^0
  In2 : Inport  Port=2  OutDataType=sfix(16)  OutScaling=2^0
  In3 : Inport  Port=3  OutDataType=sfix(16)  OutScaling=2^0
  Output1 : Sum  Inputs=|+-+  OutDataType=sfix(16)  OutScaling=2^0  SaturateOnIntegerOverflow=on  InputSameDT=on
  RO : RelationalOperator  Operator=<  LogicOutDataTypeMode=boolean
  Switch : Switch  Criteria=u2 > Threshold
  Out1 : Outport  OutDataType=sfix(16)  OutScaling=2^0
  wires:
  In3/1 -> Output1/3
  Output1/1 -> Switch/1
  RO/1 -> Switch/2
  Switch/1 -> Out1/1
  In2/1 -> RO/1, Output1/1, Switch/3  "U(k)"
  In1/1 -> RO/2, Output1/2

== system MIL_Test/Test Data/Feature generation/Generate timed limited decrease/Subsystem/Subsystem31 ==
  In1 : Inport  OutDataType=sfix(16)  OutScaling=2^0
  In2 : Inport  Port=2  OutDataType=sfix(16)  OutScaling=2^0
  In3 : Inport  Port=3  OutDataType=sfix(16)  OutScaling=2^0
  Output1 : Sum  Inputs=|+-+  OutDataType=sfix(16)  OutScaling=2^0  SaturateOnIntegerOverflow=on  InputSameDT=on
  RO : RelationalOperator  Operator=<  LogicOutDataTypeMode=boolean
  Switch : Switch  Criteria=u2 > Threshold
  Out1 : Outport  OutDataType=sfix(16)  OutScaling=2^0
  wires:
  In3/1 -> Output1/3
  Output1/1 -> Switch/1
  RO/1 -> Switch/2
  Switch/1 -> Out1/1
  In2/1 -> RO/1, Output1/1, Switch/3  "U(k)"
  In1/1 -> RO/2, Output1/2

== system MIL_Test/Test Data/Feature generation/Generate timed limited decrease/Subsystem/Subsystem32 ==
  In1 : Inport  OutDataType=sfix(16)  OutScaling=2^0
  In2 : Inport  Port=2  OutDataType=sfix(16)  OutScaling=2^0
  In3 : Inport  Port=3  OutDataType=sfix(16)  OutScaling=2^0
  Output1 : Sum  Inputs=|+-+  OutDataType=sfix(16)  OutScaling=2^0  SaturateOnIntegerOverflow=on  InputSameDT=on
  RO : RelationalOperator  Operator=<  LogicOutDataTypeMode=boolean
  Switch : Switch  Criteria=u2 > Threshold
  Out1 : Outport  OutDataType=sfix(16)  OutScaling=2^0
  wires:
  In3/1 -> Output1/3
  Output1/1 -> Switch/1
  RO/1 -> Switch/2
  Switch/1 -> Out1/1
  In2/1 -> RO/1, Output1/1, Switch/3  "U(k)"
  In1/1 -> RO/2, Output1/2

== system MIL_Test/Test Data/Feature generation/Generate timed limited decrease/Subsystem/Subsystem33 ==
  In1 : Inport  OutDataType=sfix(16)  OutScaling=2^0
  In2 : Inport  Port=2  OutDataType=sfix(16)  OutScaling=2^0
  In3 : Inport  Port=3  OutDataType=sfix(16)  OutScaling=2^0
  Output1 : Sum  Inputs=|+-+  OutDataType=sfix(16)  OutScaling=2^0  SaturateOnIntegerOverflow=on  InputSameDT=on
  RO : RelationalOperator  Operator=<  LogicOutDataTypeMode=boolean
  Switch : Switch  Criteria=u2 > Threshold
  Out1 : Outport  OutDataType=sfix(16)  OutScaling=2^0
  wires:
  In3/1 -> Output1/3
  Output1/1 -> Switch/1
  RO/1 -> Switch/2
  Switch/1 -> Out1/1
  In2/1 -> RO/1, Output1/1, Switch/3  "U(k)"
  In1/1 -> RO/2, Output1/2

== system MIL_Test/Test Data/Feature generation/Generate timed limited decrease/Subsystem/Subsystem34 ==
  In1 : Inport  OutDataType=sfix(16)  OutScaling=2^0
  In2 : Inport  Port=2  OutDataType=sfix(16)  OutScaling=2^0
  In3 : Inport  Port=3  OutDataType=sfix(16)  OutScaling=2^0
  Output1 : Sum  Inputs=|+-+  OutDataType=sfix(16)  OutScaling=2^0  SaturateOnIntegerOverflow=on  InputSameDT=on
  RO : RelationalOperator  Operator=<  LogicOutDataTypeMode=boolean
  Switch : Switch  Criteria=u2 > Threshold
  Out1 : Outport  OutDataType=sfix(16)  OutScaling=2^0
  wires:
  In3/1 -> Output1/3
  Output1/1 -> Switch/1
  RO/1 -> Switch/2
  Switch/1 -> Out1/1
  In2/1 -> RO/1, Output1/1, Switch/3  "U(k)"
  In1/1 -> RO/2, Output1/2

== system MIL_Test/Test Data/Feature generation/Generate timed limited decrease/Subsystem/Subsystem35 ==
  In1 : Inport  OutDataType=sfix(16)  OutScaling=2^0
  In2 : Inport  Port=2  OutDataType=sfix(16)  OutScaling=2^0
  In3 : Inport  Port=3  OutDataType=sfix(16)  OutScaling=2^0
  Output1 : Sum  Inputs=|+-+  OutDataType=sfix(16)  OutScaling=2^0  SaturateOnIntegerOverflow=on  InputSameDT=on
  RO : RelationalOperator  Operator=<  LogicOutDataTypeMode=boolean
  Switch : Switch  Criteria=u2 > Threshold
  Out1 : Outport  OutDataType=sfix(16)  OutScaling=2^0
  wires:
  In3/1 -> Output1/3
  Output1/1 -> Switch/1
  RO/1 -> Switch/2
  Switch/1 -> Out1/1
  In2/1 -> RO/1, Output1/1, Switch/3  "U(k)"
  In1/1 -> RO/2, Output1/2

== system MIL_Test/Test Data/Feature generation/Generate timed limited decrease/Subsystem/Subsystem36 ==
  In1 : Inport  OutDataType=sfix(16)  OutScaling=2^0
  In2 : Inport  Port=2  OutDataType=sfix(16)  OutScaling=2^0
  In3 : Inport  Port=3  OutDataType=sfix(16)  OutScaling=2^0
  Output1 : Sum  Inputs=|+-+  OutDataType=sfix(16)  OutScaling=2^0  SaturateOnIntegerOverflow=on  InputSameDT=on
  RO : RelationalOperator  Operator=<  LogicOutDataTypeMode=boolean
  Switch : Switch  Criteria=u2 > Threshold
  Out1 : Outport  OutDataType=sfix(16)  OutScaling=2^0
  wires:
  In3/1 -> Output1/3
  Output1/1 -> Switch/1
  RO/1 -> Switch/2
  Switch/1 -> Out1/1
  In2/1 -> RO/1, Output1/1, Switch/3  "U(k)"
  In1/1 -> RO/2, Output1/2

== system MIL_Test/Test Data/Feature generation/Generate timed limited decrease/Subsystem/Subsystem37 ==
  In1 : Inport  OutDataType=sfix(16)  OutScaling=2^0
  In2 : Inport  Port=2  OutDataType=sfix(16)  OutScaling=2^0
  In3 : Inport  Port=3  OutDataType=sfix(16)  OutScaling=2^0
  Output1 : Sum  Inputs=|+-+  OutDataType=sfix(16)  OutScaling=2^0  SaturateOnIntegerOverflow=on  InputSameDT=on
  RO : RelationalOperator  Operator=<  LogicOutDataTypeMode=boolean
  Switch : Switch  Criteria=u2 > Threshold
  Out1 : Outport  OutDataType=sfix(16)  OutScaling=2^0
  wires:
  In3/1 -> Output1/3
  Output1/1 -> Switch/1
  RO/1 -> Switch/2
  Switch/1 -> Out1/1
  In2/1 -> RO/1, Output1/1, Switch/3  "U(k)"
  In1/1 -> RO/2, Output1/2

== system MIL_Test/Test Data/Feature generation/Generate timed limited decrease/Subsystem/Subsystem38 ==
  In1 : Inport  OutDataType=sfix(16)  OutScaling=2^0
  In2 : Inport  Port=2  OutDataType=sfix(16)  OutScaling=2^0
  In3 : Inport  Port=3  OutDataType=sfix(16)  OutScaling=2^0
  Output1 : Sum  Inputs=|+-+  OutDataType=sfix(16)  OutScaling=2^0  SaturateOnIntegerOverflow=on  InputSameDT=on
  RO : RelationalOperator  Operator=<  LogicOutDataTypeMode=boolean
  Switch : Switch  Criteria=u2 > Threshold
  Out1 : Outport  OutDataType=sfix(16)  OutScaling=2^0
  wires:
  In3/1 -> Output1/3
  Output1/1 -> Switch/1
  RO/1 -> Switch/2
  Switch/1 -> Out1/1
  In2/1 -> RO/1, Output1/1, Switch/3  "U(k)"
  In1/1 -> RO/2, Output1/2

== system MIL_Test/Test Data/Feature generation/Generate timed limited decrease/Subsystem/Subsystem39 ==
  In1 : Inport  OutDataType=sfix(16)  OutScaling=2^0
  In2 : Inport  Port=2  OutDataType=sfix(16)  OutScaling=2^0
  In3 : Inport  Port=3  OutDataType=sfix(16)  OutScaling=2^0
  Output1 : Sum  Inputs=|+-+  OutDataType=sfix(16)  OutScaling=2^0  SaturateOnIntegerOverflow=on  InputSameDT=on
  RO : RelationalOperator  Operator=<  LogicOutDataTypeMode=boolean
  Switch : Switch  Criteria=u2 > Threshold
  Out1 : Outport  OutDataType=sfix(16)  OutScaling=2^0
  wires:
  In3/1 -> Output1/3
  Output1/1 -> Switch/1
  RO/1 -> Switch/2
  Switch/1 -> Out1/1
  In2/1 -> RO/1, Output1/1, Switch/3  "U(k)"
  In1/1 -> RO/2, Output1/2

== system MIL_Test/Test Data/Feature generation/Generate timed limited decrease/Subsystem/Subsystem4 ==
  In1 : Inport  OutDataType=sfix(16)  OutScaling=2^0
  In2 : Inport  Port=2  OutDataType=sfix(16)  OutScaling=2^0
  In3 : Inport  Port=3  OutDataType=sfix(16)  OutScaling=2^0
  Output1 : Sum  Inputs=|+-+  OutDataType=sfix(16)  OutScaling=2^0  SaturateOnIntegerOverflow=on  InputSameDT=on
  RO : RelationalOperator  Operator=<  LogicOutDataTypeMode=boolean
  Switch : Switch  Criteria=u2 > Threshold
  Out1 : Outport  OutDataType=sfix(16)  OutScaling=2^0
  wires:
  In3/1 -> Output1/3
  Output1/1 -> Switch/1
  RO/1 -> Switch/2
  Switch/1 -> Out1/1
  In2/1 -> RO/1, Output1/1, Switch/3  "U(k)"
  In1/1 -> RO/2, Output1/2
